simulink library "Lib_Model"  (R2024b)
settings: Solver=VariableStepAuto  StartTime=0.0  StopTime=10.0  RelTol=1e-3
undefined symbols (not defined in the file): DiscIntNeverNeededParam
settings Model: Creator=HHI  LastModifiedBy=HHI

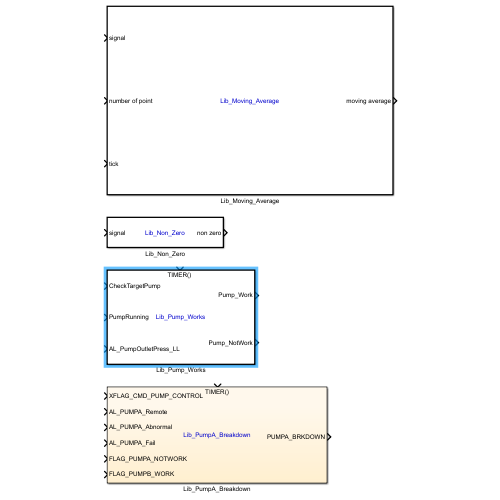
[thumbnail: Simulink's stored preview of the top-level diagram]
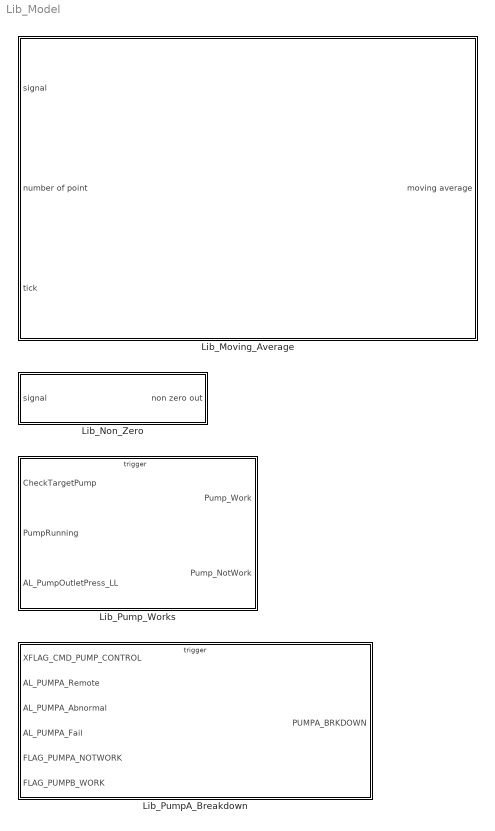
== system Lib_Model ==
  Lib_Moving_Average : Subsystem  TreatAsAtomicUnit=on  RTWFcnName=Moving_Avearge
      settings: RTWFcnNameOpts=User specified
      mask Display:
      | color('blue');
      | disp('Lib_Moving_Average');
      | 
      | color('black');
      | port_label('input', 1, 'signal');
      | port_label('input', 2, 'number of point');
      | port_label('input', 3, 'tick');
      | port_label('output', 1, 'moving average');
  Lib_Non_Zero : Subsystem  TreatAsAtomicUnit=on  RTWFcnName=Non_Zero
      settings: RTWFcnNameOpts=User specified
      mask Display:
      | color('blue');
      | disp('Lib_Non_Zero');
      | 
      | color('black');
      | port_label('input', 1, 'signal');
      | port_label('output', 1, 'non zero');
  Lib_PumpA_Breakdown : Stateflow chart  TreatAsAtomicUnit=on  RTWFcnName=PumpA_Breakdown
      settings: RTWSystemCode=Reusable function  RTWFcnNameOpts=User specified
  Lib_Pump_Works : Subsystem  TreatAsAtomicUnit=on  RTWFcnName=Pump_Works
      settings: RTWFcnNameOpts=User specified
      mask Display:
      | color('blue');
      | disp('Lib_Pump_Works');
      | 
      | color('black');
      | port_label('Trigger', 'TIMER()')
      | 
      | port_label('input', 1, 'CheckTargetPump');
      | port_label('input', 2, 'PumpRunning');
      | port_label('input', 3, 'AL_PumpOutletPress_LL');
      | port_label('output', 1, 'Pump_Work');
      | port_label('output', 2, 'Pump_NotWork');

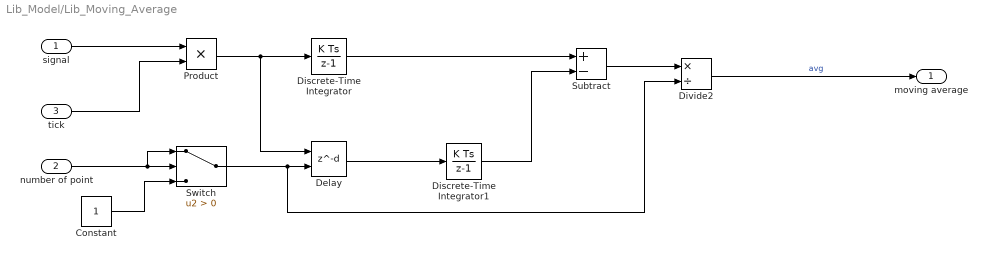
== system Lib_Model/Lib_Moving_Average ==
  signal : Inport  OutDataTypeStr=single  PortDimensions=1
  number of point : Inport  Port=2  OutDataTypeStr=single  PortDimensions=1
  tick : Inport  Port=3  OutDataTypeStr=single  PortDimensions=1
  Constant : Constant  OutDataTypeStr=single  LockScale=on
  Delay : Delay  DelayLengthSource=Input port
      settings: InputPortMap=u0,p1
  Discrete-Time Integrator : DiscreteIntegrator  SampleTime=-1  ICPrevOutput=DiscIntNeverNeededParam  ICPrevScaledInput=DiscIntNeverNeededParam
  Discrete-Time Integrator1 : DiscreteIntegrator  SampleTime=-1  ICPrevOutput=DiscIntNeverNeededParam  ICPrevScaledInput=DiscIntNeverNeededParam
  Divide2 : Product  Inputs=*/
  Product : Product
  Subtract : Sum  Inputs=+-
  Switch : Switch  Criteria=u2 > Threshold  SaturateOnIntegerOverflow=off  InputSameDT=off
  moving average : Outport  OutDataTypeStr=single  PortDimensions=1
  wires:
  Product/1 -> Discrete-Time Integrator/1, Delay/1
  Discrete-Time Integrator/1 -> Subtract/1
  Discrete-Time Integrator1/1 -> Subtract/2
  tick/1 -> Product/2
  signal/1 -> Product/1
  number of point/1 -> Switch/2, Switch/1
  Switch/1 -> Delay/2, Divide2/2
  Delay/1 -> Discrete-Time Integrator1/1
  Constant/1 -> Switch/3
  Divide2/1 -> moving average/1  "avg"
  Subtract/1 -> Divide2/1

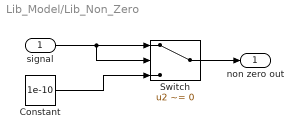
== system Lib_Model/Lib_Non_Zero ==
  signal : Inport  OutDataTypeStr=single
  Constant : Constant  Value=1e-10  OutDataTypeStr=single
  Switch : Switch  Criteria=u2 ~= 0  SaturateOnIntegerOverflow=off  InputSameDT=off
  non zero out : Outport  OutDataTypeStr=single  PortDimensions=1
  wires:
  signal/1 -> Switch/2, Switch/1
  Constant/1 -> Switch/3
  Switch/1 -> non zero out/1

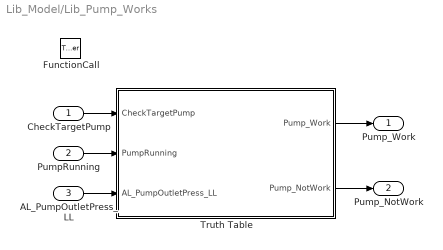
== system Lib_Model/Lib_Pump_Works ==
  CheckTargetPump : Inport  OutDataTypeStr=boolean  PortDimensions=1
  PumpRunning : Inport  Port=2  OutDataTypeStr=boolean  PortDimensions=1
  AL_PumpOutletPress_LL : Inport  Port=3  OutDataTypeStr=boolean  PortDimensions=1
  FunctionCall : TriggerPort  TriggerType=function-call  VariantControl=(inherit)  PortDimensions=1
  Truth Table : Truth Table  TreatAsAtomicUnit=on
  Pump_Work : Outport  OutDataTypeStr=boolean  PortDimensions=1  InitialOutput=0
  Pump_NotWork : Outport  Port=2  OutDataTypeStr=boolean  PortDimensions=1  InitialOutput=0
  wires:
  PumpRunning/1 -> Truth Table/2(PumpRunning)
  Truth Table/1(Pump_Work) -> Pump_Work/1
  AL_PumpOutletPress_LL/1 -> Truth Table/3(AL_PumpOutletPress_LL)
  Truth Table/2(Pump_NotWork) -> Pump_NotWork/1
  CheckTargetPump/1 -> Truth Table/1(CheckTargetPump)

== stateflow chart Lib_Model/Lib_PumpA_Breakdown ==
  settings: sampleTime=SamplingTime  executeAtInitialization=1
  state CHECK_FLAG
    state CHECK_FLAG_PUMPA__BRKDOWN [parallel]
      settings: executionOrder=1
      state FLAG_OFF
        en:
        PUMPA_BRKDOWN = 0;
      state FLAG_ON
        en:
        PUMPA_BRKDOWN = 1;
      (default) -> FLAG_OFF
      FLAG_OFF -> FLAG_ON [order 2] : [FLAG_PUMPA_NOTWORK == 1]
          | // [MASTER PUMP == A ...
          | // || CDI_AFOSupplypumpRunning == 1 ...
          | // || AL_FOSupplyOutletPress_LL == 1]
      FLAG_OFF -> FLAG_ON [order 1] : [AL_PUMPA_Remote == 1 ...
          | || AL_PUMPA_Abnormal == 1 ...
          | || AL_PUMPA_Fail == 1]
      (junction 44) -> FLAG_OFF [order 1] : [XFLAG_CMD_PUMP_CONTROL == 0 ...
          | || FLAG_PUMPB_WORK == 1]
          | // [MASTER PUMP == B ...
          | // || CDI_BFOSupplypumpRunning == 1 ...
          | // || AL_FOSupplyOutletPress_LL == 0]
      (junction 44) -> (junction 46) [order 2]
      FLAG_ON -> (junction 44) : [!(AL_PUMPA_Remote == 1 ...
          | || AL_PUMPA_Abnormal == 1 ...
          | || AL_PUMPA_Fail == 1)]
      (junction 46) -> FLAG_ON
  (default) -> CHECK_FLAG
  data: XFLAG_CMD_PUMP_CONTROL input boolean size=1; AL_PUMPA_Remote input boolean size=1; PUMPA_BRKDOWN output boolean size=1 =0; AL_PUMPA_Abnormal input boolean size=1; AL_PUMPA_Fail input boolean size=1; FLAG_PUMPA_NOTWORK input boolean; FLAG_PUMPB_WORK input boolean
  events: TIMER input FUNCTION_CALL_EVENT

== matlab function Lib_Model/Lib_Pump_Works/Truth Table ==
  data: CheckTargetPump input boolean size=1; Pump_Work output boolean size=1 =0; PumpRunning input boolean size=1; AL_PumpOutletPress_LL input boolean size=1; Pump_NotWork output boolean size=1 =0
function [Pump_Work, Pump_NotWork] = fcn(CheckTargetPump, PumpRunning, AL_PumpOutletPress_LL)

aVarTruthTableCondition_1 = false;
aVarTruthTableCondition_2 = false;


% Target Pump Runnung

aVarTruthTableCondition_1 = logical((CheckTargetPump == 1) && (PumpRunning == 1));

% PumpOutletPress_LL Alarm Active

aVarTruthTableCondition_2 = logical(AL_PumpOutletPress_LL);

if (aVarTruthTableCondition_1 && ~aVarTruthTableCondition_2)
    aFcnTruthTableAction_1();
elseif (aVarTruthTableCondition_1 && aVarTruthTableCondition_2)
    aFcnTruthTableAction_2();
else % Default
    aFcnTruthTableAction_3();
end

function aFcnTruthTableAction_1()

% Pump is working normally

Pump_Work = true;
Pump_NotWork = false;

function aFcnTruthTableAction_2()

% Pump is not working normally.

Pump_Work = false;
Pump_NotWork = true;

function aFcnTruthTableAction_3()

% N/A

Pump_Work = false;
Pump_NotWork = false;
